simulink model "control_block"  (R2020b)
settings: Solver=VariableStepAuto  StartTime=0.0  StopTime=10.0  RelTol=1e-3
settings Model: Creator=Palo  LastModifiedBy=Palo

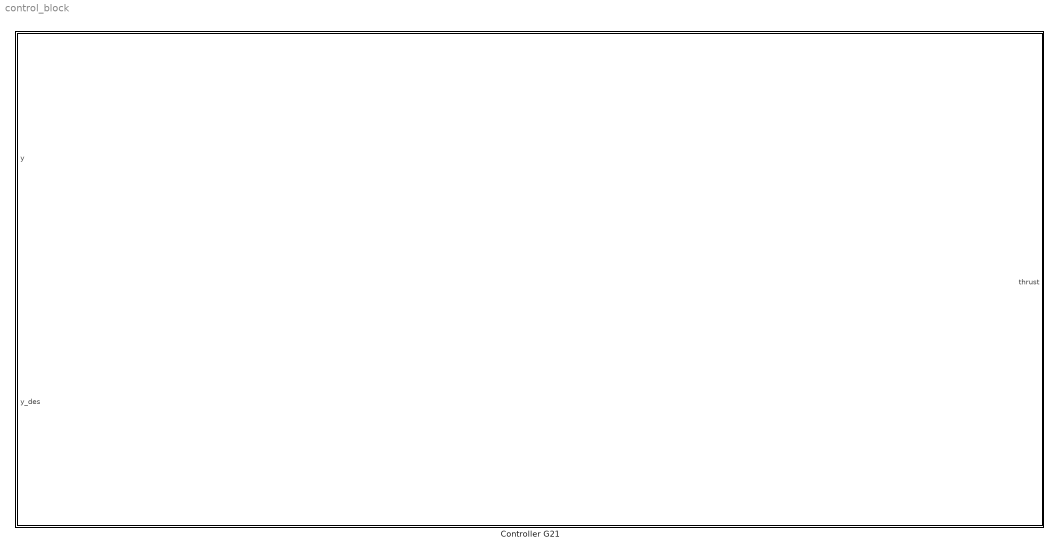
== system control_block ==
  Controller G21 : Subsystem

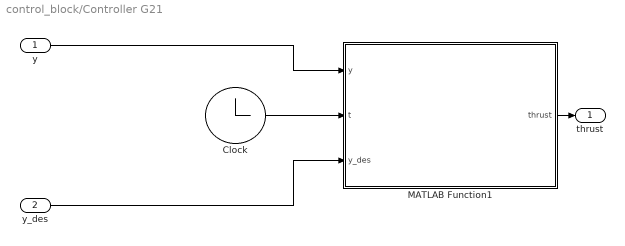
== system control_block/Controller G21 ==
  y : Inport
  y_des : Inport  Port=2
  Clock : Clock
  MATLAB Function1 : MATLAB Function  TreatAsAtomicUnit=on
  thrust : Outport
  wires:
  y_des/1 -> MATLAB Function1/3(y_des)
  MATLAB Function1/1(thrust) -> thrust/1
  y/1 -> MATLAB Function1/1(y)
  Clock/1 -> MATLAB Function1/2(t)

== matlab function control_block/Controller G21/MATLAB Function1 ==
  settings: updateMethod=DISCRETE
  data: y input; thrust output; t input; y_des input
function thrust = lqr_controller(y, t, y_des)
    persistent y_prev y_prev_prev t_prev v_est thrust_est
    
    %% Persistent vars initialisation
    if isempty(y_prev)
        y_prev = -1;
        y_prev_prev = 0;
        t_prev = -1;
        v_est = 0;
        thrust_est = 0;
        
        thrust = 0;
        return
    end
    
    %% Constants
    K = [0.951141031602812, 17.5829247933687];
    drop_velocity = -4;
    drop_y = 0.1;
    
    %% LQR Calc
    err = y_des - y;
    v = (3*y - 4*y_prev + y_prev_prev) / (2*(t - t_prev)); % 2nd order backwards diff

    y_prev_prev = y_prev;
    y_prev = y;
    t_prev = t;

    v_est = 0.12*(v - v_est) + v_est;
    v = v_est;
    
    thrust = -K*[v; -err];

    thrust_est = 0.5*(thrust - thrust_est) + thrust_est;
    thrust = thrust_est;
    
    %% Drop condition
    if y_des < drop_y && y < 0.6 && v < drop_velocity
        % Reduce velocity so as to not hit too hard
        % Max drop velocity should be -3
        %thrust = drop_thrust;
        v_err = v - drop_velocity;
        thrust = -v_err;
    end
end
